simulink model "mod_6Dof"  (R2023b)
settings: Solver=FixedStepAuto  StartTime=0.0  StopTime=10  FixedStep=0.01  MaxStep=0.02  RelTol=1e-5  AbsTol=1e-7
values from neighbouring files (symbols this model uses):
  sample_time = 0.01    [DOF6.m]
undefined symbols (not defined in the file or in its folder): deg, rad, s
libraries: aerolibconvert2 x2, shared6dof x1
settings Model: Creator=The MathWorks, Inc.  LastModifiedBy=kbs_s
settings SolverCC: AutoScaleAbsTol=off  AlgebraicLoopSolver=TrustRegion
settings DataIOCC: SaveFormat=Array  SaveOutput=off  ReturnWorkspaceOutputs=off
settings OptimizationCC: DefaultParameterBehavior=Inlined  OptimizeBlockIOStorage=off  ReuseModelBlockBuffer=off  ExpressionDepthLimit=2147483647  ZeroExternalMemoryAtStartup=off  ZeroInternalMemoryAtStartup=off  InitFltsAndDblsToZero=on  LifeSpan=inf  OptimizeDataStoreBuffers=off  BusAssignmentInplaceUpdate=off
settings DebuggingCC: SaveWithParameterizedLinksMsg=none  MultiTaskCondExecSysMsg=none  SigSpecEnsureSampleTimeMsg=none  FcnCallInpInsideContextMsg=warning  UnconnectedInputMsg=warning  UnconnectedOutputMsg=warning  UnconnectedLineMsg=warning  UniqueDataStoreMsg=error  StateNameClashWarn=warning  StrictBusMsg=ErrorOnBusTreatedAsVector  SFUnexpectedBacktrackingDiag=warning  SFNoUnconditionalDefaultTransitionDiag=warning  SFExecutionAtInitializationDiag=none  ArithmeticOperatorsInVariantConditions=warning
settings HardwareCC: ProdBitPerPointer=32  ProdLargestAtomicFloat=None  ProdIntDivRoundTo=Undefined  ProdEndianess=Unspecified  ProdWordSize=32  ProdHWDeviceType=32-bit Generic  TargetBitPerPointer=64  TargetBitPerSizeT=64  TargetBitPerPtrDiffT=64  TargetLongLongMode=on  TargetIntDivRoundTo=Zero  TargetEndianess=LittleEndian  TargetWordSize=64  TargetHWDeviceType=MATLAB Host  ProdEqTarget=off
settings ModelReferenceCC: EnableRefExpFcnMdlSchedulingChecks=on  PropagateSignalLabelsOutOfModel=off
settings SFSimCC: SimUseLocalCustomCode=off  CustomCodeUndefinedFunction=UseInterfaceOnly
settings RTWCC: GenerateMakefile=off  TemplateMakefile=grt_vc.tmf  GenerateReport=on  RTWUseLocalCustomCode=off  BuildConfiguration=Debug  LaunchReport=on  TargetLang=C++
settings CodeAppCC: ForceParamTrailComments=on  MATLABSourceComments=on  EnableCustomComments=on
settings GRTTargetCC: TargetFcnLib=ansi_tfl_tmw.mat  TargetLangStandard=C++11 (ISO)  CombineSignalStateStructs=on  CodeInterfacePackaging=C++ class  SupportVariableSizeSignals=on  MultiInstanceErrorCode=Warning
settings ConfigComp: CovMetricSettings=d  CovSaveCumulativeToWorkspaceVar=on  CovSaveSingleToWorkspaceVar=on  CovExternalEMLEnable=off

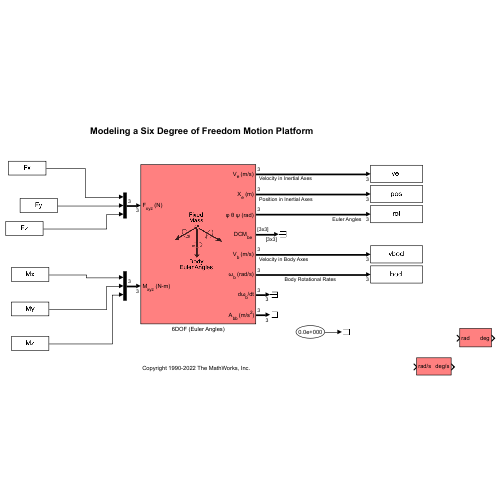
[thumbnail: Simulink's stored preview of the top-level diagram]
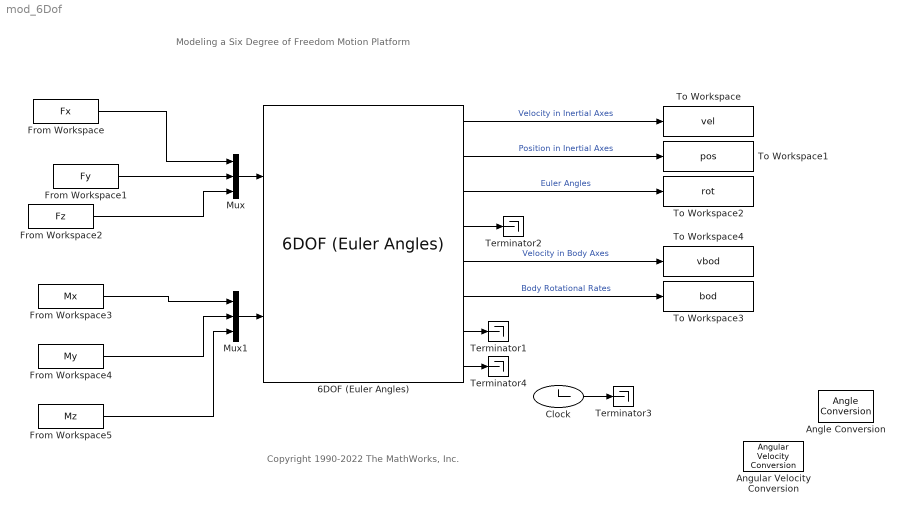
== system mod_6Dof ==
  note: Modeling a Six Degree of Freedom Motion Platform
  note: Copyright 1990-2022 The MathWorks, Inc.
  6DOF (Euler Angles) : shared6dof/6DOF (Euler Angles)  units=Metric (MKS)  mtype=Fixed  rep=Euler Angles  xme_0=[0 0 0]  Vm_0=[0 0 0]  eul_0=[0 0 0]  pm_0=[0 0 0]  mass_0=1.0  mass_e=0.5  mass_f=2.0  inertia=eye(3)  inertia_e=eye(3)  inertia_f=2*eye(3)  k_quat=1.0  vre_flag=on  abi_flag=off  aMode=0  xme_statename=''  Vm_statename=''  eul_statename=''  quat_statename=''  pm_statename=''  mass_statename=''
  Angle Conversion : aerolibconvert2/Angle Conversion  IU=rad  OU=deg
  Angular Velocity Conversion : aerolibconvert2/Angular Velocity Conversion  IU=rad/s  OU=deg/s
  Clock : Clock
      settings: Decimation=100
  From Workspace : FromWorkspace  VariableName=Fx  SampleTime=sample_time
  From Workspace1 : FromWorkspace  VariableName=Fy  SampleTime=sample_time
  From Workspace2 : FromWorkspace  VariableName=Fz  SampleTime=sample_time
  From Workspace3 : FromWorkspace  VariableName=Mx  SampleTime=sample_time
  From Workspace4 : FromWorkspace  VariableName=My  SampleTime=sample_time
  From Workspace5 : FromWorkspace  VariableName=Mz  SampleTime=sample_time
  Mux : Mux  Inputs=3
  Mux1 : Mux  Inputs=3
  Terminator{1..4} (4 alike) : Terminator
  To Workspace : ToWorkspace  VariableName=vel  SaveFormat=Timeseries  SampleTime=-1
  To Workspace1 : ToWorkspace  VariableName=pos  SaveFormat=Timeseries  SampleTime=-1
  To Workspace2 : ToWorkspace  VariableName=rot  SaveFormat=Timeseries  SampleTime=-1
  To Workspace3 : ToWorkspace  VariableName=bod  SaveFormat=Timeseries  SampleTime=-1
  To Workspace4 : ToWorkspace  VariableName=vbod  SaveFormat=Timeseries  SampleTime=-1
  wires:
  Clock/1 -> Terminator3/1
  Mux1/1 -> 6DOF (Euler Angles)/2
  From Workspace5/1 -> Mux1/3
  From Workspace4/1 -> Mux1/2
  From Workspace3/1 -> Mux1/1
  Mux/1 -> 6DOF (Euler Angles)/1
  From Workspace1/1 -> Mux/2
  From Workspace2/1 -> Mux/3
  From Workspace/1 -> Mux/1
  6DOF (Euler Angles)/4 -> Terminator2/1
  6DOF (Euler Angles)/7 -> Terminator1/1
  6DOF (Euler Angles)/5 -> To Workspace4/1  "Velocity in Body Axes"
  6DOF (Euler Angles)/1 -> To Workspace/1  "Velocity in Inertial Axes"
  6DOF (Euler Angles)/2 -> To Workspace1/1  "Position in Inertial Axes"
  6DOF (Euler Angles)/3 -> To Workspace2/1  "Euler Angles"
  6DOF (Euler Angles)/6 -> To Workspace3/1  "Body Rotational Rates"
  6DOF (Euler Angles)/8 -> Terminator4/1
